simulink model "SimulinkProject - Kopie (2)"  (R2025b)
settings: Solver=ode5  StartTime=0.0  StopTime=150  FixedStep=1/3200  RelTol=1e-3
model workspace (MAT data in the model file):
  radius = 100
libraries: simulink x2, eeGeneralControl x2, simulink_extras x2
settings Model: Creator=Fabian  LastModifiedBy=Fabian

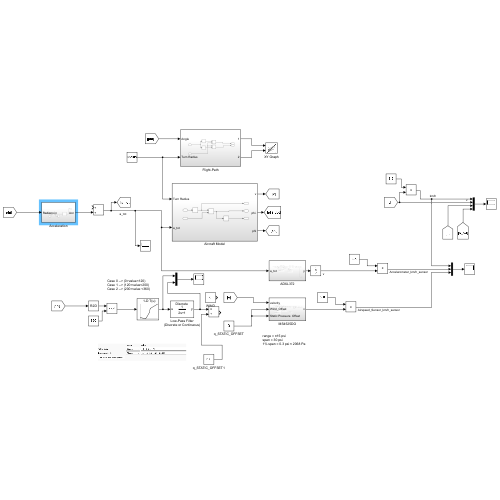
[thumbnail: Simulink's stored preview of the top-level diagram]
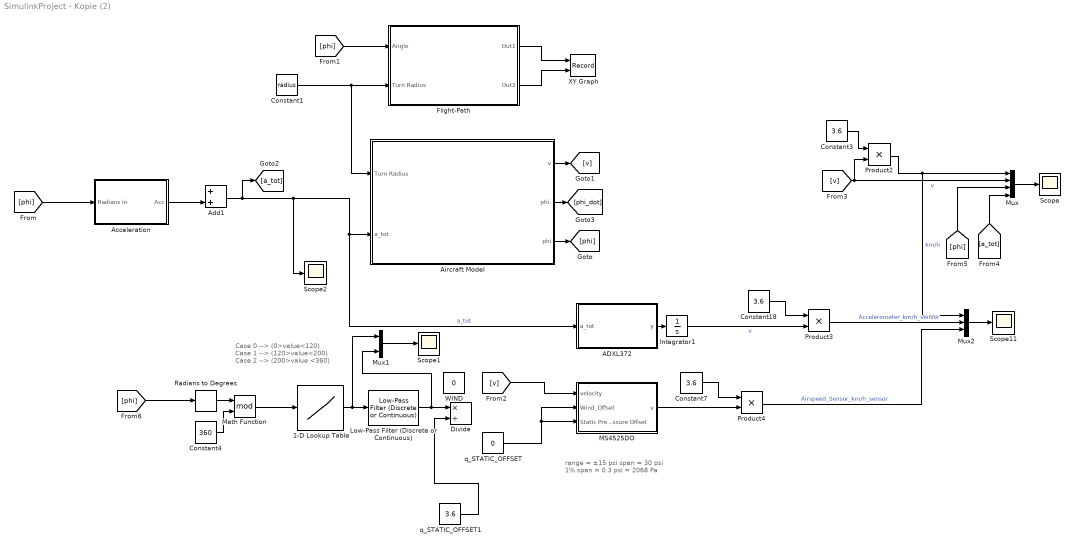
== system SimulinkProject - Kopie (2) ==
  note: range = ±15 psi
      | span = 30 psi
      | 1% span = 0.3 psi ≈ 2068 Pa
  note: Case 0 --> (0>value<120)
      | Case 1 --> (120>value<200)
      | Case 2 --> (200>value <360)
  1-D Lookup Table : Lookup_n-D  NumberOfTableDimensions=1  BreakpointsForDimension1=[0 110 130 190 210 360]  Table=[30 20 30 60 90 120]  InterpMethod=Linear Lagrange  InternalRulePriority=Speed  RndMeth=Simplest
  ADXL372 : Subsystem
  Acceleration : Subsystem
  Add1 : Sum
  Aircraft Model : Subsystem
  Constant1 : Constant  Value=radius
  Constant18 : Constant  Value=3.6
  Constant3 : Constant  Value=3.6
  Constant4 : Constant  Value=360
  Constant7 : Constant  Value=3.6
  Divide : Product  Inputs=*/
  Flight-Path : Subsystem
  Integrator1 : Integrator  InitialCondition=13
  Low-Pass Filter (Discrete or Continuous) : eeGeneralControl/Low-Pass Filter (Discrete or Continuous)  K=1  T=2  B=inf  A=-inf  init_option=Inherited from block input  x0=0  Ts=-1
  MS4525DO : Subsystem
  Math Function : Math  Operator=mod
  Mux : Mux
  Mux1 : Mux  Inputs=2
  Mux2 : Mux  Inputs=3
  Product2 : Product
  Product3 : Product
  Product4 : Product
  Radians to Degrees : simulink_extras/Transformations/Radians to Degrees
  Scope{,1..2,11} (4 alike) : Scope
      Scope settings: ActiveDisplayYMinimum=-26.414661447647582  ActiveDisplayYMaximum=14.251796061942557
      Scope1 settings: ActiveDisplayYMinimum=7.5000170386444847  ActiveDisplayYMaximum=132.49993809872853  DataLoggingVariableName=ScopeData2
      Scope11 settings: ActiveDisplayYMinimum=518.97191220786715  ActiveDisplayYMaximum=530.05750876519267  DataLoggingVariableName=ScopeData11
      Scope2 settings: ActiveDisplayYMinimum=-4.125  ActiveDisplayYMaximum=7.1250000000000009  DataLoggingVariableName=ScopeData3
  WIND : Constant  Value=0
  XY Graph : Record  NumPorts=2.0  FileSettingsInternal="{\"entries\":[{\"content\":{\"excelSettings\":{\"content\":{},\"type\":\"Streamout.ExcelSettings\"},\"parquetSettings\":{\"content\":{},\"type\":\"Streamout.ParquetSettings\"}},\"type\":\"Streamout.FileSettingStorage\",\"uuid\":\"\"}],\"packageUris\":[\"http:\\/\\/schema.mathworks.com\\/mf0\\/streamout_blocks\\/R2020a\"],\"version\":\"1.0\"}"  FrameSettings=[0, 0]  Layout=[1 1]  SignalsInternal="{\"entries\":[{\"content\":{\"signals\":[{\"content\":{\"blockPath\":[],\"dimensions\":[1],\"domain\":\"\",\"lineColor\":\"#a2142f\",\"plots\":[ 1 ],\"port\":1,\"sid\":[\"\"],\"signalID\":1,\"signalName\":\"Flight-Path:1\"},\"type\":\"RecordBlkView.Signal\",\"uuid\":\"\"},{\"content\":{\"blockPath\":[],\"dimensions\":[1],\"domain\":\"\",\"lineColor\":\"#139fff\",\"plots\":[ 1 ],\"port\":2,\"sid\":[\"\"],\"signalID\":2,\"signalName\":\"Flight-Path:2\"},\"type\":\"RecordBlkView.Signal\",\"uuid\":\"\"}]},\"type\":\"RecordBlkView.InputSignals\",\"uuid\":\"\"}],\"packageUris\":[\"http:\\/\\/schema.mathworks.com\\/mf0\\/streamout_blocks\\/R2020a\"],\"version\":\"1.0\"}"  VisualizationBindings="{\"xyplotplugin\":{\"info\":[{\"series\":[{\"bindingParametersList\":[{\"parameter\":\"X-Axis\",\"signalID\":1,\"signalName\":\"Flight-Path:1\"},{\"parameter\":\"Y-Axis\",\"signalID\":2,\"signalName\":\"Flight-Path:2\"}],\"seriesID\":0}],\"subplotID\":1}]}}"  CompatibilityTag=XY
  q_STATIC_OFFSET : Constant  Value=0
  q_STATIC_OFFSET1 : Constant  Value=3.6
  wires:
  Add1/1 -> ADXL372/1(a_tot), Aircraft Model/2(a_tot), Scope2/1, [a_tot]  "a_tot"
  Constant1/1 -> Flight-Path/2(Turn Radius), Aircraft Model/1(Turn Radius)
  Product2/1 -> Mux2/1, Mux/1  "km/h"
  Constant18/1 -> Product3/1
  Integrator1/1 -> Product3/2  "v"
  Mux2/1 -> Scope11/1
  Product3/1 -> Mux2/2  "Accelerometer_km/h_sensor"
  ADXL372/1(y) -> Integrator1/1
  Acceleration/1(Acc) -> Add1/2
  [phi] -> Acceleration/1(Radians in)
  Constant7/1 -> Product4/1
  Product4/1 -> Mux2/3  "Airspeed_Sensor_km/h_sensor"
  [v] -> MS4525DO/1(velocity)
  q_STATIC_OFFSET/1 -> MS4525DO/2(Wind_Offset), MS4525DO/3(Static Pressure Offset)
  MS4525DO/1(v) -> Product4/2
  [phi] -> Flight-Path/1(Angle)
  Flight-Path/1(Out1) -> XY Graph/1
  Flight-Path/2(Out2) -> XY Graph/2
  [v] -> Product2/2, Mux/2  "v"
  [a_tot] -> Mux/4
  [phi] -> Mux/3
  Aircraft Model/1(v) -> [v]
  Aircraft Model/2(phi.) -> [phi_dot]
  Aircraft Model/3(phi) -> [phi]
  Constant3/1 -> Product2/1
  Mux/1 -> Scope/1
  Radians to Degrees/1 -> Math Function/1
  Math Function/1 -> 1-D Lookup Table/1
  Constant4/1 -> Math Function/2
  1-D Lookup Table/1 -> Mux1/1, Low-Pass Filter (Discrete or Continuous)/1
  q_STATIC_OFFSET1/1 -> Divide/2
  [phi] -> Radians to Degrees/1
  Low-Pass Filter (Discrete or Continuous)/1 -> Mux1/2, Divide/1
  Mux1/1 -> Scope1/1

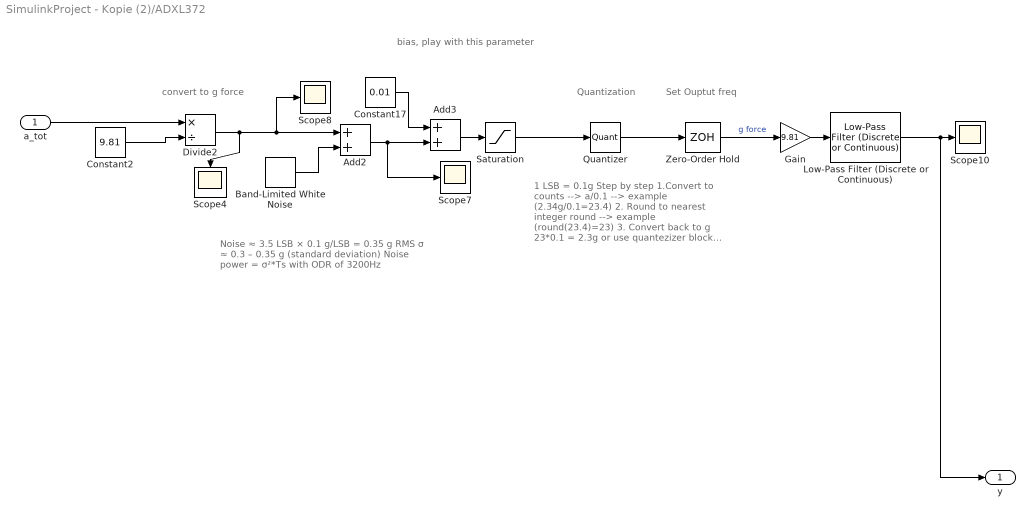
== system SimulinkProject - Kopie (2)/ADXL372 ==
  note: convert to g force
  note: Noise ≈ 3.5 LSB × 0.1 g/LSB = 0.35 g RMS
      | σ ≈ 0.3 – 0.35 g (standard deviation)
      | Noise power = σ²*Ts
      | with ODR of 3200Hz
  note: bias, play with this parameter
  note: Quantization
  note: 1 LSB = 0.1g
      | Step by step
      |
      | 1.Convert to counts
      | --> a/0.1 --> example (2.34g/0.1=23.4)
      | 2. Round to nearest integer
      | round --> example (round(23.4)=23)
      | 3. Convert back to g
      | 23*0.1 = 2.3g
      |
      | or use quantezizer block with 0.1
  note: Set Ouptut freq
  a_tot : Inport
  Add2 : Sum
  Add3 : Sum
  Band-Limited White Noise : simulink/Sources/Band-Limited White Noise  Cov=((0.35)^2)*(1/3200)  Ts=1/3200  seed=[23341]
  Constant17 : Constant  Value=0.01
  Constant2 : Constant  Value=9.81
  Divide2 : Product  Inputs=*/
  Gain : Gain  Gain=9.81
  Low-Pass Filter (Discrete or Continuous) : eeGeneralControl/Low-Pass Filter (Discrete or Continuous)  K=1  T=1/(2*pi*10)  B=inf  A=-inf  init_option=Inherited from block input  x0=0  Ts=1/3200
  Quantizer : Quantizer  QuantizationInterval=0.1
  Saturation : Saturate  UpperLimit=200  LowerLimit=-200
  Scope{4,7..8,10} (4 alike) : Scope
      Scope10 settings: ActiveDisplayYMinimum=-5.375623541068566  ActiveDisplayYMaximum=9.3751831580889746  DataLoggingVariableName=ScopeData10
      Scope4 settings: ActiveDisplayYMinimum=-8.7987661112898756  ActiveDisplayYMaximum=16.470735842466532  DataLoggingVariableName=ScopeData4
      Scope7 settings: ActiveDisplayYMinimum=-2.1194574766866134  ActiveDisplayYMaximum=2.6082539117818122  DataLoggingVariableName=ScopeData7
      Scope8 settings: ActiveDisplayYMinimum=-0.3058103975535168  ActiveDisplayYMaximum=0.71355759429153931  DataLoggingVariableName=ScopeData8
  Zero-Order Hold : ZeroOrderHold  SampleTime=1/3200
  y : Outport
  wires:
  Constant2/1 -> Divide2/2
  Add3/1 -> Saturation/1
  Saturation/1 -> Quantizer/1
  Divide2/1 -> Add2/1, Scope8/1, Scope4/1
  Gain/1 -> Low-Pass Filter (Discrete or Continuous)/1
  Add2/1 -> Scope7/1, Add3/2
  Constant17/1 -> Add3/1
  Band-Limited White Noise/1 -> Add2/2
  Quantizer/1 -> Zero-Order Hold/1
  Zero-Order Hold/1 -> Gain/1  "g force"
  Low-Pass Filter (Discrete or Continuous)/1 -> y/1, Scope10/1
  a_tot/1 -> Divide2/1

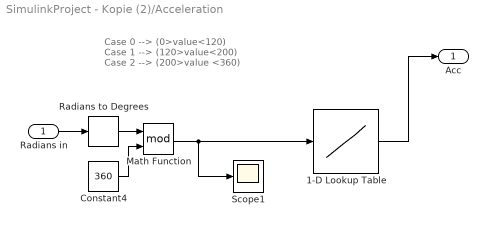
== system SimulinkProject - Kopie (2)/Acceleration ==
  note: Case 0 --> (0>value<120)
      | Case 1 --> (120>value<200)
      | Case 2 --> (200>value <360)
  Radians in : Inport
  1-D Lookup Table : Lookup_n-D  NumberOfTableDimensions=1  BreakpointsForDimension1=[0 110 130 190 210 360]  Table=[-3 -3 6 6 4 4]  InterpMethod=Linear Lagrange  InternalRulePriority=Speed  RndMeth=Simplest
  Constant4 : Constant  Value=360
  Math Function : Math  Operator=mod
  Radians to Degrees : simulink_extras/Transformations/Radians to Degrees
  Scope1 : Scope
      settings: ActiveDisplayYMinimum=-47.332509505790171  ActiveDisplayYMaximum=913.02258838484045
  Acc : Outport
  wires:
  Radians to Degrees/1 -> Math Function/1
  Constant4/1 -> Math Function/2
  Math Function/1 -> Scope1/1, 1-D Lookup Table/1
  Radians in/1 -> Radians to Degrees/1
  1-D Lookup Table/1 -> Acc/1

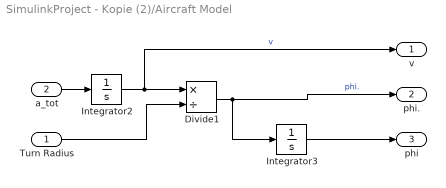
== system SimulinkProject - Kopie (2)/Aircraft Model ==
  Turn Radius : Inport
  a_tot : Inport  Port=2
  Divide1 : Product  Inputs=*/
  Integrator2 : Integrator  InitialCondition=13
  Integrator3 : Integrator  InitialCondition=pi
  v : Outport
  phi. : Outport  Port=2
  phi : Outport  Port=3
  wires:
  Divide1/1 -> phi./1, Integrator3/1  "phi."
  Integrator3/1 -> phi/1
  Integrator2/1 -> v/1, Divide1/1  "v"
  Turn Radius/1 -> Divide1/2
  a_tot/1 -> Integrator2/1

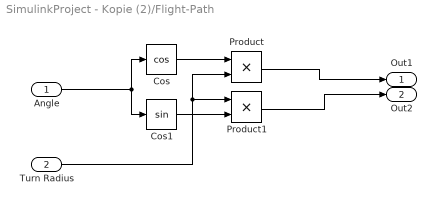
== system SimulinkProject - Kopie (2)/Flight-Path ==
  Angle : Inport
  Turn Radius : Inport  Port=2
  Cos : Trigonometry  Operator=cos
  Cos1 : Trigonometry
  Product : Product
  Product1 : Product
  Out1 : Outport
  Out2 : Outport  Port=2
  wires:
  Cos1/1 -> Product1/2
  Turn Radius/1 -> Product/2, Product1/1
  Angle/1 -> Cos1/1, Cos/1
  Cos/1 -> Product/1
  Product1/1 -> Out2/1
  Product/1 -> Out1/1

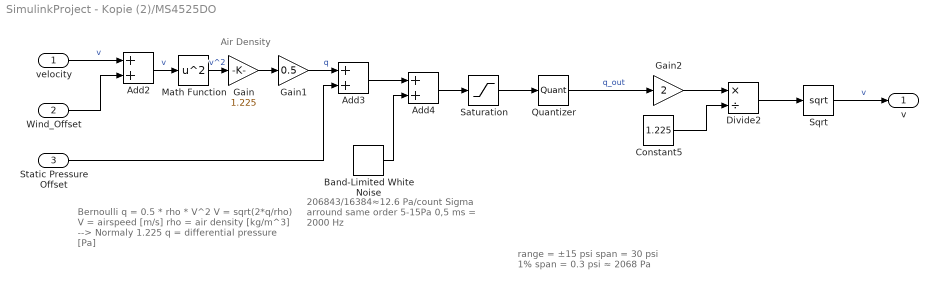
== system SimulinkProject - Kopie (2)/MS4525DO ==
  note: Bernoulli
      | q = 0.5 * rho * V^2
      | V = sqrt(2*q/rho)
      |
      | V = airspeed [m/s]
      | rho = air density [kg/m^3] --> Normaly 1.225
      | q = differential pressure [Pa]
  note: Air Density
  note: 206843/16384​≈12.6 Pa/count
      | Sigma arround same order 5-15Pa
      |
      | 0,5 ms = 2000 Hz
  note: range = ±15 psi
      | span = 30 psi
      | 1% span = 0.3 psi ≈ 2068 Pa
  velocity : Inport
  Wind_Offset : Inport  Port=2
  Static Pressure Offset : Inport  Port=3
  Add2 : Sum
  Add3 : Sum
  Add4 : Sum
  Band-Limited White Noise : simulink/Sources/Band-Limited White Noise  Cov=((10)^2)*(1/3200)  Ts=1/3200  seed=[23341]
  Constant5 : Constant  Value=1.225
  Divide2 : Product  Inputs=*/
  Gain : Gain  Gain=1.225
  Gain1 : Gain  Gain=0.5
  Gain2 : Gain  Gain=2
  Math Function : Math  Operator=square
  Quantizer : Quantizer  QuantizationInterval=12.6
  Saturation : Saturate  UpperLimit=103421  LowerLimit=-103421
  Sqrt : Sqrt
  v : Outport
  wires:
  Add3/1 -> Add4/1
  Divide2/1 -> Sqrt/1
  Add2/1 -> Math Function/1  "v"
  Saturation/1 -> Quantizer/1
  Math Function/1 -> Gain/1  "v^2"
  Gain/1 -> Gain1/1
  Gain1/1 -> Add3/1  "q"
  Add4/1 -> Saturation/1
  Gain2/1 -> Divide2/1
  Wind_Offset/1 -> Add2/2
  Constant5/1 -> Divide2/2
  Quantizer/1 -> Gain2/1  "q_out"
  Band-Limited White Noise/1 -> Add4/2
  velocity/1 -> Add2/1  "v"
  Static Pressure Offset/1 -> Add3/2
  Sqrt/1 -> v/1  "v"
